simulink model "taskBasedWalking_legacy"  (Simulink 8.3)
settings: Solver=FixedStepDiscrete  StartTime=0.0  StopTime=Config.t_end  FixedStep=Config.t_step  RelTol=1e-3
InitFcn:
  | cd(fileparts(which(bdroot)));
  | initTaskBasedWalking;
StopFcn:
  | cd(fileparts(which(bdroot)));
  | stopTaskBasedWalking;
undefined symbols (not defined in the file): biasVectorConstraint_feet, Config, ConstraintMatrix_feet, DiscIntNeverNeededParam, Gains, ROBOT_DOF, Sat
libraries: WBToolboxLibrary x78
(part 2 of 3)

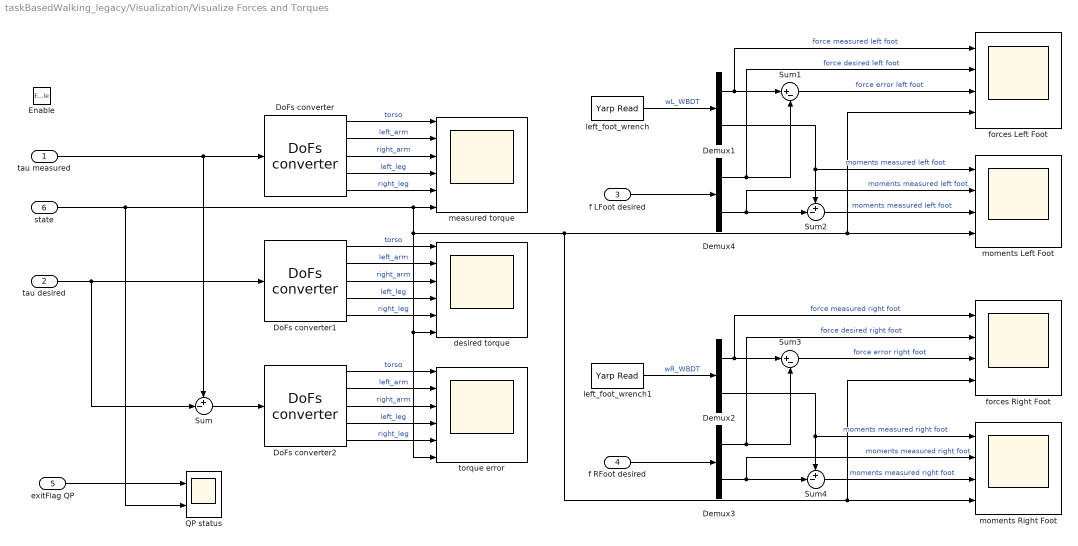
== system taskBasedWalking_legacy/Visualization/Visualize Forces and Torques ==
  tau measured : Inport
  tau desired : Inport  Port=2
  f LFoot desired : Inport  Port=3
  f RFoot desired : Inport  Port=4
  exitFlag QP : Inport  Port=5
  state : Inport  Port=6
  Enable : EnablePort
  Demux{1..4} (4 alike) : Demux  Outputs=[3;3]
  DoFs converter : WBToolboxLibrary/Utilities/DoFs converter  yarp2WBIOption=From YARP to WBI
  DoFs converter1 : WBToolboxLibrary/Utilities/DoFs converter  yarp2WBIOption=From YARP to WBI
  DoFs converter2 : WBToolboxLibrary/Utilities/DoFs converter  yarp2WBIOption=From YARP to WBI
  QP status : Scope  NumInputPorts=2
      settings: TimeRange=auto  MaxDataPoints=5000  SaveName=exitFlagQP_DATA  YMin=-1.00000~0.75  YMax=1.00000~3.25  SampleTime=-1
  Sum : Sum  Inputs=+-|
  Sum1 : Sum  Inputs=|+-
  Sum2 : Sum  Inputs=+-|
  Sum3 : Sum  Inputs=|+-
  Sum4 : Sum  Inputs=+-|
  desired torque : Scope  NumInputPorts=6
      settings: TimeRange=14  ShowLegends=on  MaxDataPoints=5000  SaveName=tauDes_DATA  YMin=-29.31633~-6.97567~-8.31868~-17.81518~-20.85132~0.75  YMax=21.22105~7.45092~10.09722~31.90811~36.21162~3.25  SampleTime=-1
  forces Left Foot : Scope  NumInputPorts=4
      settings: TimeRange=40  MaxDataPoints=5000  SaveName=LFoot_forces_DATA  YMin=-94.50547~-90.33374~-124.32192~0.75  YMax=380.58154~375.05705~119.64102~3.25  SampleTime=-1
  forces Right Foot : Scope  NumInputPorts=4
      settings: TimeRange=40  MaxDataPoints=5000  SaveName=RFoot_forces_DATA  YMin=-51.60497~-22.1975~-34.93363~0.9  YMax=197.58058~186.84107~13.61516~1.1  SampleTime=-1
  left_foot_wrench : WBToolboxLibrary/Utilities/Yarp Read  portName=Ports.LEFT_FOOT_EXT_WRENCH  signalSize=6  timeout=0.5  blocking=off  timestamp=off  autoconnect=on  errorOnConnection=on
  left_foot_wrench1 : WBToolboxLibrary/Utilities/Yarp Read  portName=Ports.RIGHT_FOOT_EXT_WRENCH  signalSize=6  timeout=0.5  blocking=off  timestamp=off  autoconnect=on  errorOnConnection=on
  measured torque : Scope  NumInputPorts=6
      settings: TimeRange=14  ShowLegends=on  MaxDataPoints=5000  SaveName=tauMeas_DATA  YMin=-11.47679~-4.18596~-4.23181~-18.73707~-21.78999~0.75  YMax=12.06319~6.82355~7.49283~33.43238~33.30445~3.25  SampleTime=-1
  moments Left Foot : Scope  NumInputPorts=4
      settings: TimeRange=40  ShowLegends=on  MaxDataPoints=5000  SaveName=LFoot_moments_DATA  YMin=-9.62259~-10.62436~-12.71673~0.75  YMax=14.01039~14.13793~13.77201~3.25  SampleTime=-1
  moments Right Foot : Scope  NumInputPorts=4
      settings: TimeRange=40  MaxDataPoints=5000  SaveName=RFoot_moments_DATA  YMin=-32.91586~-23.80001~-19.34028~0.75  YMax=21.19597~19.42571~23.95955~3.25  SampleTime=-1
  torque error : Scope  NumInputPorts=6
      settings: TimeRange=14  ShowLegends=on  MaxDataPoints=5000  SaveName=tauErr_DATA  YMin=-24.82167~-15.35375~-17.84626~-32.8437~-37.60868~0.75  YMax=19.17022~15.52326~18.81152~24.48279~21.81289~3.25  SampleTime=-1
  wires:
  Sum2/1 -> moments Left Foot/3  "moments measured left foot"
  state/1 -> QP status/2, torque error/6, desired torque/6, forces Right Foot/4, moments Right Foot/4, forces Left Foot/4, moments Left Foot/4, measured torque/6
  DoFs converter1/2 -> desired torque/2  "left_arm"
  Demux4/1 -> forces Left Foot/2, Sum1/2  "force desired left foot"
  DoFs converter2/1 -> torque error/1  "torso"
  DoFs converter1/4 -> desired torque/4  "left_leg"
  Demux4/2 -> moments Left Foot/2, Sum2/2  "moments measured left foot"
  DoFs converter/1 -> measured torque/1  "torso"
  DoFs converter2/3 -> torque error/3  "right_arm"
  f RFoot desired/1 -> Demux3/1
  DoFs converter1/1 -> desired torque/1  "torso"
  Sum4/1 -> moments Right Foot/3  "moments measured right foot"
  tau desired/1 -> Sum/2, DoFs converter1/1
  Demux2/1 -> forces Right Foot/1, Sum3/1  "force measured right foot"
  DoFs converter2/2 -> torque error/2  "left_arm"
  Sum3/1 -> forces Right Foot/3  "force error right foot"
  DoFs converter/5 -> measured torque/5  "right_leg"
  DoFs converter2/5 -> torque error/5  "right_leg"
  exitFlag QP/1 -> QP status/1
  left_foot_wrench/1 -> Demux1/1  "wL_WBDT"
  DoFs converter1/3 -> desired torque/3  "right_arm"
  Demux3/1 -> forces Right Foot/2, Sum3/2  "force desired right foot"
  f LFoot desired/1 -> Demux4/1
  Sum1/1 -> forces Left Foot/3  "force error left foot"
  tau measured/1 -> Sum/1, DoFs converter/1
  DoFs converter1/5 -> desired torque/5  "right_leg"
  DoFs converter/2 -> measured torque/2  "left_arm"
  DoFs converter/3 -> measured torque/3  "right_arm"
  Demux3/2 -> moments Right Foot/2, Sum4/2  "moments measured right foot"
  Sum/1 -> DoFs converter2/1
  Demux1/1 -> forces Left Foot/1, Sum1/1  "force measured left foot"
  DoFs converter/4 -> measured torque/4  "left_leg"
  Demux1/2 -> moments Left Foot/1, Sum2/1  "moments measured left foot"
  left_foot_wrench1/1 -> Demux2/1  "wR_WBDT"
  DoFs converter2/4 -> torque error/4  "left_leg"
  Demux2/2 -> moments Right Foot/1, Sum4/1  "moments measured right foot"

== system taskBasedWalking_legacy/Visualization/Visualize Gain Scheduling ==
  Kp_CoM : Inport
  Kd_CoM : Inport  Port=2
  Kp_LFoot : Inport  Port=3
  Kd_LFoot : Inport  Port=4
  Kp_RFoot : Inport  Port=5
  Kd_RFoot : Inport  Port=6
  Kp_rot_task : Inport  Port=7
  Kd_rot_task : Inport  Port=8
  impedances : Inport  Port=9
  dampings : Inport  Port=10
  state : Inport  Port=11
  Enable : EnablePort
  DoFs converter1 : WBToolboxLibrary/Utilities/DoFs converter  yarp2WBIOption=From YARP to WBI
  DoFs converter4 : WBToolboxLibrary/Utilities/DoFs converter  yarp2WBIOption=From YARP to WBI
  joint position gains : Scope  NumInputPorts=6
      settings: TimeRange=auto  MaxDataPoints=5000  SaveName=impedances_DATA  YMin=-10~-10~-10~-10~-10~-10  YMax=10~10~10~10~10~10  SampleTime=-1
  joint velocity gains : Scope  NumInputPorts=6
      settings: TimeRange=auto  MaxDataPoints=5000  SaveName=dampings_DATA  YMin=-1.00000~-1.00000~-1.00000~-1.00000~-1.00000~0.9  YMax=1.00000~1.00000~1.00000~1.00000~1.00000~1.1  SampleTime=-1
  orient gains rot task : Scope  NumInputPorts=2
      settings: TimeRange=auto  MaxDataPoints=5000  SaveName=Kp_rot_task_DATA  YMin=40.00000~0.75  YMax=60.00000~3.25  SampleTime=-1
  pos gains CoM : Scope  NumInputPorts=2
      settings: TimeRange=auto  MaxDataPoints=5000  SaveName=Kp_CoM_DATA  YMin=40.00000~0.75  YMax=60.00000~3.25  SampleTime=-1
  pose gains LFoot : Scope  NumInputPorts=2
      settings: TimeRange=auto  MaxDataPoints=5000  SaveName=Kp_LFoot_DATA  YMin=-9.375~0.75  YMax=834.375~3.25  SampleTime=-1
  pose gains RFoot : Scope  NumInputPorts=2
      settings: TimeRange=auto  MaxDataPoints=5000  SaveName=Kp_RFoot_DATA  YMin=-0.15075~0.9  YMax=0.68063~1.1  SampleTime=-1
  vel gains CoM : Scope  NumInputPorts=2
      settings: TimeRange=auto  MaxDataPoints=5000  SaveName=Kd_CoM_DATA  YMin=12.3762~0.625  YMax=15.10531~4.375  SampleTime=-1
  vel gains LFoot : Scope  NumInputPorts=2
      settings: TimeRange=auto  MaxDataPoints=5000  SaveName=Kd_LFoot_DATA  YMin=0.31598~0.75  YMax=1.48634~3.25  SampleTime=-1
  vel gains RFoot : Scope  NumInputPorts=2
      settings: TimeRange=auto  MaxDataPoints=5000  SaveName=Kd_RFoot_DATA  YMin=-0.15075~0.9  YMax=0.68063~1.1  SampleTime=-1
  vel gains rot task : Scope  NumInputPorts=2
      settings: TimeRange=auto  MaxDataPoints=5000  SaveName=Kd_rot_task_DATA  YMin=-0.15075~0.9  YMax=0.68063~1.1  SampleTime=-1
  wires:
  Kp_CoM/1 -> pos gains CoM/1
  Kp_LFoot/1 -> pose gains LFoot/1
  Kp_RFoot/1 -> pose gains RFoot/1
  Kp_rot_task/1 -> orient gains rot task/1
  state/1 -> vel gains LFoot/2, pose gains LFoot/2, vel gains CoM/2, vel gains rot task/2, orient gains rot task/2, vel gains RFoot/2, joint velocity gains/6, joint position gains/6, pose gains RFoot/2, pos gains CoM/2
  Kd_CoM/1 -> vel gains CoM/1
  Kd_LFoot/1 -> vel gains LFoot/1
  Kd_RFoot/1 -> vel gains RFoot/1
  Kd_rot_task/1 -> vel gains rot task/1
  DoFs converter4/2 -> joint position gains/2  "left_arm"
  DoFs converter4/1 -> joint position gains/1  "torso"
  DoFs converter4/4 -> joint position gains/4  "left_leg"
  DoFs converter4/3 -> joint position gains/3  "right_arm"
  DoFs converter4/5 -> joint position gains/5  "right_leg"
  DoFs converter1/2 -> joint velocity gains/2  "left_arm"
  DoFs converter1/1 -> joint velocity gains/1  "torso"
  DoFs converter1/4 -> joint velocity gains/4  "left_leg"
  DoFs converter1/3 -> joint velocity gains/3  "right_arm"
  DoFs converter1/5 -> joint velocity gains/5  "right_leg"
  impedances/1 -> DoFs converter4/1
  dampings/1 -> DoFs converter1/1

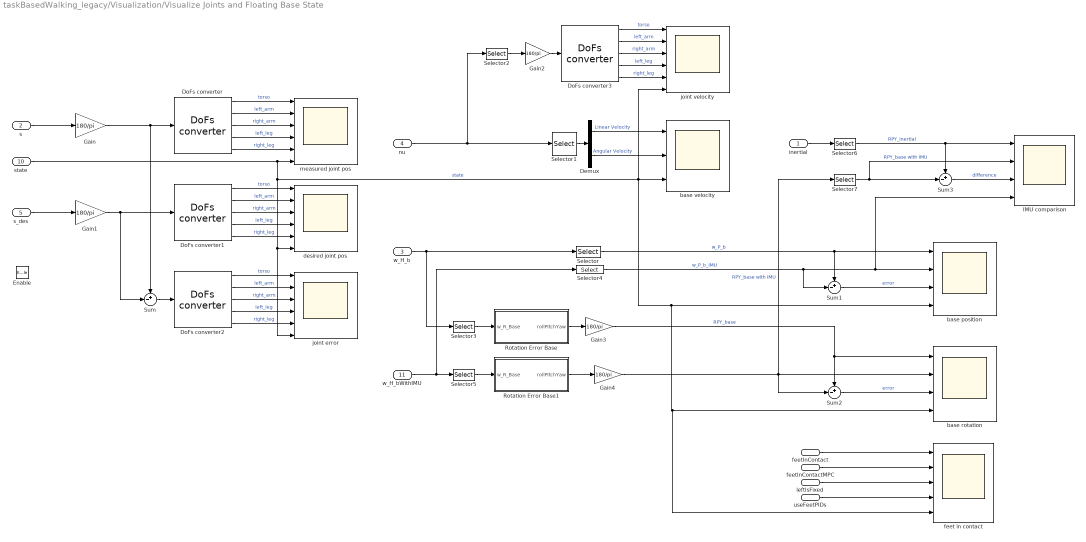
== system taskBasedWalking_legacy/Visualization/Visualize Joints and Floating Base State ==
  inertial : Inport
  s : Inport  Port=2
  w_H_b : Inport  Port=3
  nu : Inport  Port=4
  s_des : Inport  Port=5
  feetInContact : Inport  Port=6
  useFeetPIDs : Inport  Port=7
  feetInContactMPC : Inport  Port=8
  leftIsFixed : Inport  Port=9
  state : Inport  Port=10
  w_H_bWithIMU : Inport  Port=11
  Enable : EnablePort
  Demux : Demux  Outputs=2
  DoFs converter{,1..3} (4 alike) : WBToolboxLibrary/Utilities/DoFs converter  yarp2WBIOption=From YARP to WBI
  Gain{,1..4} (5 alike) : Gain  Gain=180/pi
  IMU comparison : Scope  NumInputPorts=4
      settings: TimeRange=auto  MaxDataPoints=5000  SaveToWorkspace=off  SaveName=ScopeData2  YMin=-12.46344~-15.58042~-22.96688~-0.21919  YMax=8.17339~13.72293~16.2002~0.70364  SampleTime=-1
  Rotation Error Base : Subsystem
  Rotation Error Base1 : Subsystem
  Selector : Selector  NumberOfDimensions=2  InputPortWidth=3  IndexOptions=Index vector (dialog),Index vector (dialog)  Indices=[1:3],4  OutputSizes=1,1
  Selector1 : Selector  InputPortWidth=ROBOT_DOF+6  IndexOptions=Index vector (dialog)  Indices=[1:6]  OutputSizes=1
  Selector2 : Selector  InputPortWidth=ROBOT_DOF+6  IndexOptions=Index vector (dialog)  Indices=[7:ROBOT_DOF+6]  OutputSizes=1
  Selector3 : Selector  NumberOfDimensions=2  InputPortWidth=3  IndexOptions=Index vector (dialog),Index vector (dialog)  Indices=[1:3],[1:3]  OutputSizes=1,1
  Selector4 : Selector  NumberOfDimensions=2  InputPortWidth=3  IndexOptions=Index vector (dialog),Index vector (dialog)  Indices=[1:3],4  OutputSizes=1,1
  Selector5 : Selector  NumberOfDimensions=2  InputPortWidth=3  IndexOptions=Index vector (dialog),Index vector (dialog)  Indices=[1:3],[1:3]  OutputSizes=1,1
  Selector6 : Selector  InputPortWidth=12  IndexOptions=Index vector (dialog)  Indices=[1:2]  OutputSizes=1
  Selector7 : Selector  InputPortWidth=3  IndexOptions=Index vector (dialog)  Indices=[1:2]  OutputSizes=1
  Sum{,1..3} (4 alike) : Sum  Inputs=+-|
  base position : Scope  NumInputPorts=4
      settings: TimeRange=auto  MaxDataPoints=5000  SaveName=basePos_DATA  YMin=-0.22398~-0.21941~-0.00771~0.75  YMax=0.95033~0.93824~0.00949~3.25  SampleTime=-1
  base rotation : Scope  NumInputPorts=4
      settings: TimeRange=auto  MaxDataPoints=5000  SaveName=BaseRotation_DATA  YMin=-224.99475~-224.99475~-4.20767~0.75  YMax=224.99655~224.99655~2.37208~3.25  SampleTime=-1
  base velocity : Scope  NumInputPorts=3
      settings: TimeRange=auto  ShowLegends=on  MaxDataPoints=5000  SaveName=baseVel_DATA  YMin=-0.22618~-0.79944~0.75  YMax=0.42394~0.82635~3.25  SampleTime=-1
  desired joint pos : Scope  NumInputPorts=6
      settings: TimeRange=auto  ShowLegends=on  MaxDataPoints=5000  SaveName=jointDes_DATA  YMin=-6.59451~-23.74816~-24.05925~-41.17118~-41.50525~0.75  YMax=12.61384~48.08227~47.96861~18.71413~18.81596~3.25  SampleTime=-1
  feet in contact : Scope  NumInputPorts=5
      settings: TimeRange=auto  ShowLegends=on  MaxDataPoints=5000  SaveName=feetInContact_DATA  YMin=0.9~0.9~-1.00000~-0.125~0.9  YMax=1.1~1.1~1.00000~1.125~1.1  SampleTime=-1
  joint error : Scope  NumInputPorts=6
      settings: TimeRange=auto  ShowLegends=on  MaxDataPoints=5000  SaveName=jointErr_DATA  YMin=-13.39791~-5.05479~-5.63796~-13.82698~-9.31683~0.75  YMax=10.2644~7.99929~9.10191~9.60583~15.76566~3.25  SampleTime=-1
  joint velocity : Scope  NumInputPorts=6
      settings: TimeRange=auto  MaxDataPoints=5000  SaveName=jointVel_DATA  YMin=-65.10651~-223.32925~-75.18237~-29.76616~-17.38591~0.9  YMax=57.73467~97.18392~97.27593~28.94218~48.25756~1.1  SampleTime=-1
  measured joint pos : Scope  NumInputPorts=6
      settings: TimeRange=auto  MaxDataPoints=5000  SaveName=jointMeas_DATA  YMin=-3.77381~-21.81821~-14.09343~-38.97066~-38.66716~0.9  YMax=13.63956~37.00685~38.07115~10.81813~10.33885~1.1  SampleTime=-1
  wires:
  DoFs converter1/2 -> desired joint pos/2  "left_arm"
  DoFs converter/5 -> measured joint pos/5  "right_leg"
  DoFs converter2/1 -> joint error/1  "torso"
  DoFs converter/4 -> measured joint pos/4  "left_leg"
  DoFs converter/2 -> measured joint pos/2  "left_arm"
  s/1 -> Gain/1
  DoFs converter1/1 -> desired joint pos/1  "torso"
  DoFs converter1/4 -> desired joint pos/4  "left_leg"
  DoFs converter1/3 -> desired joint pos/3  "right_arm"
  DoFs converter/3 -> measured joint pos/3  "right_arm"
  DoFs converter2/5 -> joint error/5  "right_leg"
  DoFs converter2/2 -> joint error/2  "left_arm"
  DoFs converter/1 -> measured joint pos/1  "torso"
  s_des/1 -> Gain1/1
  DoFs converter1/5 -> desired joint pos/5  "right_leg"
  DoFs converter2/4 -> joint error/4  "left_leg"
  Sum/1 -> DoFs converter2/1
  DoFs converter2/3 -> joint error/3  "right_arm"
  DoFs converter3/5 -> joint velocity/5  "right_leg"
  DoFs converter3/1 -> joint velocity/1  "torso"
  DoFs converter3/4 -> joint velocity/4  "left_leg"
  DoFs converter3/3 -> joint velocity/3  "right_arm"
  DoFs converter3/2 -> joint velocity/2  "left_arm"
  nu/1 -> Selector2/1, Selector1/1
  w_H_b/1 -> Selector3/1, Selector/1
  Gain/1 -> Sum/1, DoFs converter/1
  Gain1/1 -> Sum/2, DoFs converter1/1
  Gain2/1 -> DoFs converter3/1
  Selector/1 -> base position/1, Sum1/1  "w_P_b"
  Selector2/1 -> Gain2/1
  state/1 -> measured joint pos/6, feet in contact/5, base rotation/4, base position/4, base velocity/3, joint velocity/6, joint error/6, desired joint pos/6  "state"
  Selector1/1 -> Demux/1
  feetInContact/1 -> feet in contact/1
  Rotation Error Base/1(rollPitchYaw) -> Gain3/1
  Gain3/1 -> Sum2/1, base rotation/1  "RPY_base"
  feetInContactMPC/1 -> feet in contact/2
  leftIsFixed/1 -> feet in contact/3
  useFeetPIDs/1 -> feet in contact/4
  Selector3/1 -> Rotation Error Base/1(w_R_Base)
  w_H_bWithIMU/1 -> Selector4/1, Selector5/1
  Selector4/1 -> Sum1/2, IMU comparison/4, base position/2  "w_P_b_IMU"
  Selector5/1 -> Rotation Error Base1/1(w_R_Base)
  Rotation Error Base1/1(rollPitchYaw) -> Gain4/1
  Sum1/1 -> base position/3  "error"
  Gain4/1 -> Selector7/1, base rotation/2, Sum2/2  "RPY_base with IMU"
  Sum2/1 -> base rotation/3  "error"
  inertial/1 -> Selector6/1
  Selector6/1 -> Sum3/1, IMU comparison/1  "RPY_inertial"
  Sum3/1 -> IMU comparison/3  "difference"
  Selector7/1 -> IMU comparison/2, Sum3/2  "RPY_base with IMU"
  Demux/1 -> base velocity/1  "Linear Velocity"
  Demux/2 -> base velocity/2  "Angular Velocity"

== system taskBasedWalking_legacy/Visualization/Visualize Smoothing (orientation) ==
  w_R_LFoot_des : Inport
  w_R_RFoot_des : Inport  Port=2
  w_R_rot_task_des : Inport  Port=3
  w_R_LFoot : Inport  Port=4
  w_R_RFoot : Inport  Port=5
  w_R_rot_task : Inport  Port=6
  V_base : Inport  Port=7
  VDot_base : Inport  Port=8
  Enable : EnablePort
  Demux : Demux  Outputs=3
  Demux1 : Demux  Outputs=3
  Demux2 : Demux  Outputs=3
  Gain : Gain  Gain=180/pi
  Gain1 : Gain  Gain=180/pi
  Gain2 : Gain  Gain=180/pi
  Rotation Error LFoot : Scope  NumInputPorts=3
      settings: TimeRange=auto  MaxDataPoints=5000  SaveName=SmootingLFoot_error_DATA  YMin=-0.000000000000000031~0.0000000000000002~-0.00000000000000006  YMax=0.000000000000000048~0.0000000000000052~0.00000000000000012  SampleTime=-1
  Rotation Error Left Foot : Subsystem
  Rotation Error RFoot : Scope  NumInputPorts=3
      settings: TimeRange=auto  ShowLegends=on  MaxDataPoints=5000  SaveName=SmootingRFoot_error_DATA  YMin=-0.04233~-0.55929~-0.07094  YMax=0.38093~0.06214~0.041  SampleTime=-1
  Rotation Error Right Foot : Subsystem
  Rotation Error Rot Task : Subsystem
  Rotation Error Rotational Task : Scope  NumInputPorts=3
      settings: TimeRange=auto  MaxDataPoints=5000  SaveName=Smooting_rot_task_error_DATA  YMin=-0.00000000000000527~0.00000000000000017539~0.000000000000000046  YMax=-0.00000000000000477~0.00000000000000017588~0.000000000000000066  SampleTime=-1
  stability of base smoothing : Scope  NumInputPorts=2
      settings: TimeRange=auto  MaxDataPoints=5000  SaveName=smoothBaseStability_DATA  YMin=-0.00125~-0.10529  YMax=0.01038~0.0117  SampleTime=-1
  wires:
  w_R_LFoot/1 -> Rotation Error Left Foot/1(w_R_LFoot)
  w_R_LFoot_des/1 -> Rotation Error Left Foot/2(w_R_LFoot_des)
  Rotation Error Left Foot/1(rollPitchYaw) -> Gain/1
  Demux/1 -> Rotation Error LFoot/1  "roll"
  Demux/2 -> Rotation Error LFoot/2  "pitch"
  Demux/3 -> Rotation Error LFoot/3  "yaw"
  w_R_RFoot/1 -> Rotation Error Right Foot/1(w_R_RFoot)
  w_R_RFoot_des/1 -> Rotation Error Right Foot/2(w_R_RFoot_des)
  Rotation Error Right Foot/1(rollPitchYaw) -> Gain1/1
  Demux1/1 -> Rotation Error RFoot/1  "roll"
  Demux1/2 -> Rotation Error RFoot/2  "pitch"
  Demux1/3 -> Rotation Error RFoot/3  "yaw"
  w_R_rot_task/1 -> Rotation Error Rot Task/1(w_R_rot_task)
  w_R_rot_task_des/1 -> Rotation Error Rot Task/2(w_R_rot_task_des)
  Rotation Error Rot Task/1(rollPitchYaw) -> Gain2/1
  Demux2/1 -> Rotation Error Rotational Task/1  "roll"
  Demux2/2 -> Rotation Error Rotational Task/2  "pitch"
  Demux2/3 -> Rotation Error Rotational Task/3  "yaw"
  Gain/1 -> Demux/1
  Gain1/1 -> Demux1/1
  Gain2/1 -> Demux2/1
  V_base/1 -> stability of base smoothing/1
  VDot_base/1 -> stability of base smoothing/2

== system taskBasedWalking_legacy/synchronizer/GAZEBO_SYNCHRONIZER ==
  Enable : EnablePort
  Simulator Synchronizer : WBToolboxLibrary/Utilities/Simulator Synchronizer  period=Config.t_step  serverPortName='/clock/rpc'  clientPortName='/WBT_synchronizer/rpc:o'

== system taskBasedWalking_legacy/synchronizer/REAL_TIME_SYNC ==
  Enable : EnablePort
  Real Time Synchronizer : WBToolboxLibrary/Utilities/Real Time Synchronizer  period=Config.t_step

== system taskBasedWalking_legacy/Dynamics and Kinematics/Compute Dynamic and Kinematic Quantities/Jacobians and JDot_nu ==
  s : Inport
  nu_b : Inport  Port=2
  sDot : Inport  Port=3
  w_H_b : Inport  Port=4
  DotJ Nu CoM : WBToolboxLibrary/wholeBodyModel/Jacobians/DotJ Nu  frameName=Frames.COM
  DotJ Nu LFoot : WBToolboxLibrary/wholeBodyModel/Jacobians/DotJ Nu  frameName=Frames.LEFT_FOOT
  DotJ Nu RFoot : WBToolboxLibrary/wholeBodyModel/Jacobians/DotJ Nu  frameName=Frames.RIGHT_FOOT
  DotJ Nu rotational task : WBToolboxLibrary/wholeBodyModel/Jacobians/DotJ Nu  frameName=Frames.ROT_TASK_LINK
  Jacobian CoM : WBToolboxLibrary/wholeBodyModel/Jacobians/Jacobian  frameName=Frames.COM
  Jacobian LFoot : WBToolboxLibrary/wholeBodyModel/Jacobians/Jacobian  frameName=Frames.LEFT_FOOT
  Jacobian RFoot : WBToolboxLibrary/wholeBodyModel/Jacobians/Jacobian  frameName=Frames.RIGHT_FOOT
  Jacobian rotational task : WBToolboxLibrary/wholeBodyModel/Jacobians/Jacobian  frameName=Frames.ROT_TASK_LINK
  J_LFoot : Outport
  J_RFoot : Outport  Port=2
  J_CoM : Outport  Port=3
  J_rot_task : Outport  Port=4
  JDot_nu_LFoot : Outport  Port=5
  JDot_nu_RFoot : Outport  Port=6
  JDot_nu_CoM : Outport  Port=7
  JDot_nu_rot_task : Outport  Port=8
  wires:
  Jacobian CoM/1 -> J_CoM/1
  Jacobian rotational task/1 -> J_rot_task/1
  Jacobian LFoot/1 -> J_LFoot/1
  Jacobian RFoot/1 -> J_RFoot/1
  w_H_b/1 -> Jacobian RFoot/1, Jacobian LFoot/1, DotJ Nu RFoot/1, DotJ Nu LFoot/1, DotJ Nu rotational task/1, DotJ Nu CoM/1, Jacobian CoM/1, Jacobian rotational task/1
  sDot/1 -> DotJ Nu RFoot/4, DotJ Nu LFoot/4, DotJ Nu rotational task/4, DotJ Nu CoM/4
  nu_b/1 -> DotJ Nu CoM/3, DotJ Nu RFoot/3, DotJ Nu LFoot/3, DotJ Nu rotational task/3
  s/1 -> DotJ Nu RFoot/2, DotJ Nu LFoot/2, DotJ Nu rotational task/2, DotJ Nu CoM/2, Jacobian RFoot/2, Jacobian CoM/2, Jacobian rotational task/2, Jacobian LFoot/2
  DotJ Nu RFoot/1 -> JDot_nu_RFoot/1
  DotJ Nu LFoot/1 -> JDot_nu_LFoot/1
  DotJ Nu rotational task/1 -> JDot_nu_rot_task/1
  DotJ Nu CoM/1 -> JDot_nu_CoM/1

== system taskBasedWalking_legacy/Dynamics and Kinematics/Compute Dynamic and Kinematic Quantities/Mass Matrix and Bias Forces ==
  s : Inport
  nu_b : Inport  Port=2
  sDot : Inport  Port=3
  w_H_b : Inport  Port=4
  Add motors reflected inertias : Subsystem
  Get Bias Forces : WBToolboxLibrary/wholeBodyModel/Dynamics/Get Bias Forces
  Mass Matrix : WBToolboxLibrary/wholeBodyModel/Dynamics/Mass Matrix
  h(q,nu) : Outport
  M(q) : Outport  Port=2
  wires:
  w_H_b/1 -> Mass Matrix/1, Get Bias Forces/1
  s/1 -> Mass Matrix/2, Get Bias Forces/2
  sDot/1 -> Get Bias Forces/4
  nu_b/1 -> Get Bias Forces/3
  Get Bias Forces/1 -> h(q,nu)/1
  Mass Matrix/1 -> Add motors reflected inertias/1(M)
  Add motors reflected inertias/1(M_with_motor_inertia) -> M(q)/1

== system taskBasedWalking_legacy/Dynamics and Kinematics/Compute Tasks Accelerations/ComputeTasksPoseAndVelocity ==
  J_LFoot : Inport
  J_RFoot : Inport  Port=2
  J_CoM : Inport  Port=3
  J_rot_task : Inport  Port=4
  s : Inport  Port=5
  w_H_b : Inport  Port=6
  nu : Inport  Port=7
  Compose Task Pose and Velocity : MATLAB Function  TreatAsAtomicUnit=on
      settings: PermitHierarchicalResolution=ParametersOnly
  Product{,1..3} (4 alike) : Product  Multiplication=Matrix(*)
  Task position and orientation : Subsystem
  pos_vel_CoM : Outport
  pose_vel_LFoot : Outport  Port=2
  pose_vel_RFoot : Outport  Port=3
  orient_vel_rot_task : Outport  Port=4
  w_H_l_sole : Outport  Port=5
  w_H_r_sole : Outport  Port=6
  wires:
  Compose Task Pose and Velocity/3(pose_vel_RFoot) -> pose_vel_RFoot/1
  Compose Task Pose and Velocity/2(pose_vel_LFoot) -> pose_vel_LFoot/1
  Compose Task Pose and Velocity/1(pos_vel_CoM) -> pos_vel_CoM/1
  Compose Task Pose and Velocity/4(orient_vel_rot_task) -> orient_vel_rot_task/1
  nu/1 -> Product1/2, Product/2, Product2/2, Product3/2
  J_rot_task/1 -> Product3/1
  Product/1 -> Compose Task Pose and Velocity/1(vel_CoM)
  Product1/1 -> Compose Task Pose and Velocity/2(vel_LFoot)
  Product2/1 -> Compose Task Pose and Velocity/3(vel_RFoot)
  Product3/1 -> Compose Task Pose and Velocity/4(vel_rot_task)
  s/1 -> Task position and orientation/1(s)
  w_H_b/1 -> Task position and orientation/2(w_H_b)
  Task position and orientation/1(w_H_CoM) -> Compose Task Pose and Velocity/5(w_H_CoM)
  Task position and orientation/2(w_H_l_sole) -> w_H_l_sole/1, Compose Task Pose and Velocity/6(w_H_l_sole)
  Task position and orientation/3(w_H_r_sole) -> w_H_r_sole/1, Compose Task Pose and Velocity/7(w_H_r_sole)
  Task position and orientation/4(w_H_rot_task) -> Compose Task Pose and Velocity/8(w_H_rot_task)
  J_RFoot/1 -> Product2/1
  J_LFoot/1 -> Product1/1
  J_CoM/1 -> Product/1

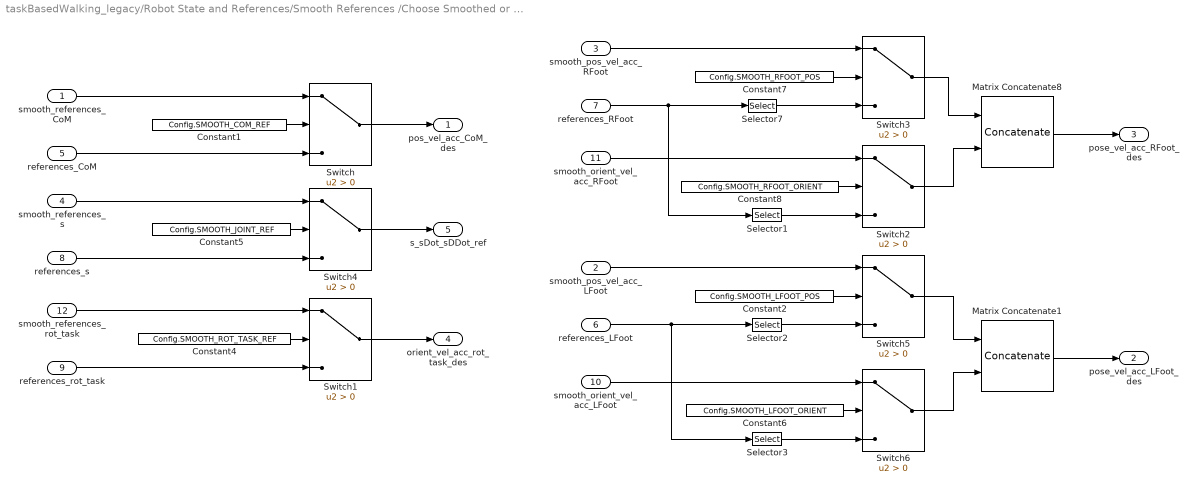
== system taskBasedWalking_legacy/Robot State and References/Smooth References /Choose Smoothed or Direct References ==
  smooth_references_CoM : Inport
  smooth_pos_vel_acc_LFoot : Inport  Port=2
  smooth_pos_vel_acc_RFoot : Inport  Port=3
  smooth_references_s : Inport  Port=4
  references_CoM : Inport  Port=5
  references_LFoot : Inport  Port=6
  references_RFoot : Inport  Port=7
  references_s : Inport  Port=8
  references_rot_task : Inport  Port=9
  smooth_orient_vel_acc_LFoot : Inport  Port=10
  smooth_orient_vel_acc_RFoot : Inport  Port=11
  smooth_references_rot_task : Inport  Port=12
  Constant1 : Constant  Value=Config.SMOOTH_COM_REF
  Constant2 : Constant  Value=Config.SMOOTH_LFOOT_POS
  Constant4 : Constant  Value=Config.SMOOTH_ROT_TASK_REF
  Constant5 : Constant  Value=Config.SMOOTH_JOINT_REF
  Constant6 : Constant  Value=Config.SMOOTH_LFOOT_ORIENT
  Constant7 : Constant  Value=Config.SMOOTH_RFOOT_POS
  Constant8 : Constant  Value=Config.SMOOTH_RFOOT_ORIENT
  Matrix Concatenate1 : Concatenate  Mode=Multidimensional array
  Matrix Concatenate8 : Concatenate  Mode=Multidimensional array
  Selector1 : Selector  NumberOfDimensions=2  InputPortWidth=ROBOT_DOF  IndexOptions=Index vector (dialog),Index vector (dialog)  Indices=[4:6],[1:5]  OutputSizes=1,1
  Selector2 : Selector  NumberOfDimensions=2  InputPortWidth=ROBOT_DOF  IndexOptions=Index vector (dialog),Index vector (dialog)  Indices=[1:3],[1:5]  OutputSizes=1,1
  Selector3 : Selector  NumberOfDimensions=2  InputPortWidth=ROBOT_DOF  IndexOptions=Index vector (dialog),Index vector (dialog)  Indices=[4:6],[1:5]  OutputSizes=1,1
  Selector7 : Selector  NumberOfDimensions=2  InputPortWidth=ROBOT_DOF  IndexOptions=Index vector (dialog),Index vector (dialog)  Indices=[1:3],[1:5]  OutputSizes=1,1
  Switch{,1..6} (7 alike) : Switch  Criteria=u2 > Threshold
  pos_vel_acc_CoM_des : Outport
  pose_vel_acc_LFoot_des : Outport  Port=2
  pose_vel_acc_RFoot_des : Outport  Port=3
  orient_vel_acc_rot_task_des : Outport  Port=4
  s_sDot_sDDot_ref : Outport  Port=5
  wires:
  Constant1/1 -> Switch/2
  Switch/1 -> pos_vel_acc_CoM_des/1
  Constant5/1 -> Switch4/2
  Switch4/1 -> s_sDot_sDDot_ref/1
  references_CoM/1 -> Switch/3
  smooth_references_CoM/1 -> Switch/1
  smooth_references_s/1 -> Switch4/1
  references_s/1 -> Switch4/3
  smooth_references_rot_task/1 -> Switch1/1
  references_rot_task/1 -> Switch1/3
  Constant4/1 -> Switch1/2
  Switch1/1 -> orient_vel_acc_rot_task_des/1
  smooth_pos_vel_acc_RFoot/1 -> Switch3/1
  Constant7/1 -> Switch3/2
  references_RFoot/1 -> Selector1/1, Selector7/1
  Selector7/1 -> Switch3/3
  smooth_orient_vel_acc_RFoot/1 -> Switch2/1
  Constant8/1 -> Switch2/2
  Selector1/1 -> Switch2/3
  Switch3/1 -> Matrix Concatenate8/1
  Switch2/1 -> Matrix Concatenate8/2
  references_LFoot/1 -> Selector3/1, Selector2/1
  Matrix Concatenate8/1 -> pose_vel_acc_RFoot_des/1
  Constant6/1 -> Switch6/2
  Matrix Concatenate1/1 -> pose_vel_acc_LFoot_des/1
  Switch5/1 -> Matrix Concatenate1/1
  Switch6/1 -> Matrix Concatenate1/2
  Constant2/1 -> Switch5/2
  Selector2/1 -> Switch5/3
  smooth_pos_vel_acc_LFoot/1 -> Switch5/1
  smooth_orient_vel_acc_LFoot/1 -> Switch6/1
  Selector3/1 -> Switch6/3

== system taskBasedWalking_legacy/Robot State and References/Smooth References /Smooth Reference Orientations ==
  w_R_LFoot_des : Inport
  w_R_RFoot_des : Inport  Port=2
  w_R_Rot_task_des : Inport  Port=3
  state : Inport  Port=4
  Compose Smoothed References : Subsystem
  Compute Smoothed Ref Orientations : Subsystem
  Constant{,1..5} (6 alike) : Constant  Value=zeros(3,1)
  smooth_orient_vel_acc_LFoot : Outport
  smooth_orient_vel_acc_RFoot : Outport  Port=2
  smooth_orient_vel_acc_Rot_task : Outport  Port=3
  wires:
  w_R_LFoot_des/1 -> Compute Smoothed Ref Orientations/1(w_R_LFoot_des)
  w_R_RFoot_des/1 -> Compute Smoothed Ref Orientations/2(w_R_RFoot_des)
  w_R_Rot_task_des/1 -> Compute Smoothed Ref Orientations/3(w_R_rot_task_des)
  Compute Smoothed Ref Orientations/3(w_R_LFoot) -> Compose Smoothed References/6(w_R_LFoot)
  Compute Smoothed Ref Orientations/2(w_R_RFoot) -> Compose Smoothed References/5(w_R_RFoot)
  Compute Smoothed Ref Orientations/1(w_R_rot_task) -> Compose Smoothed References/4(w_R_rot_task)
  Compose Smoothed References/1(orient_vel_acc_LFoot_des) -> smooth_orient_vel_acc_LFoot/1
  Compose Smoothed References/2(orient_vel_acc_RFoot_des) -> smooth_orient_vel_acc_RFoot/1
  Compose Smoothed References/3(orient_vel_acc_rot_task_des) -> smooth_orient_vel_acc_Rot_task/1
  state/1 -> Compute Smoothed Ref Orientations/4(state)
  Constant/1 -> Compose Smoothed References/1(omegaDot_LFoot)
  Constant1/1 -> Compose Smoothed References/2(omegaDot_RFoot)
  Constant2/1 -> Compose Smoothed References/3(omegaDot_rot_task)
  Constant5/1 -> Compose Smoothed References/9(omega_rot_task)
  Constant4/1 -> Compose Smoothed References/8(omega_RFoot)
  Constant3/1 -> Compose Smoothed References/7(omega_LFoot)

== system taskBasedWalking_legacy/Robot State and References/Smooth References /Smooth Reference Positions ==
  pos_CoM_des : Inport
  pos_LFoot_des : Inport  Port=2
  pos_RFoot_des : Inport  Port=3
  s_des : Inport  Port=4
  state : Inport  Port=5
  Configure Settling Times : MATLAB Function  TreatAsAtomicUnit=on
      settings: PermitHierarchicalResolution=ParametersOnly
  Matrix Concatenate1 : Concatenate  NumInputs=3  Mode=Multidimensional array  ConcatenateDimension=2
  Matrix Concatenate2 : Concatenate  NumInputs=4  Mode=Multidimensional array  ConcatenateDimension=2
  Matrix Concatenate3 : Concatenate  NumInputs=4  Mode=Multidimensional array  ConcatenateDimension=2
  Matrix Concatenate4 : Concatenate  NumInputs=3  Mode=Multidimensional array  ConcatenateDimension=2
  Minimum Jerk Trajectory Generator{,1..3} (4 alike) : WBToolboxLibrary/Utilities/Minimum Jerk Trajectory Generator  externalSettlingTime=on  settlingTime=3  sampleTime=Config.t_step  resetOnSettlingTime=off  firstDerivatives=on  secondDerivatives=on  explicitInitialValue=off
  Settling time1 : Constant  Value=zeros(3,2)
  smooth_references_CoM : Outport
  smooth_pos_vel_acc_LFoot : Outport  Port=2
  smooth_pos_vel_acc_RFoot : Outport  Port=3
  smooth_references_s : Outport  Port=4
  wires:
  Minimum Jerk Trajectory Generator2/2 -> Matrix Concatenate3/2
  pos_LFoot_des/1 -> Minimum Jerk Trajectory Generator2/1
  pos_RFoot_des/1 -> Minimum Jerk Trajectory Generator3/1
  Minimum Jerk Trajectory Generator2/3 -> Matrix Concatenate3/3
  Minimum Jerk Trajectory Generator2/1 -> Matrix Concatenate3/1
  Minimum Jerk Trajectory Generator1/3 -> Matrix Concatenate1/3
  Matrix Concatenate1/1 -> smooth_references_s/1
  Matrix Concatenate4/1 -> smooth_references_CoM/1
  Minimum Jerk Trajectory Generator1/1 -> Matrix Concatenate1/1
  pos_CoM_des/1 -> Minimum Jerk Trajectory Generator/1
  Minimum Jerk Trajectory Generator/3 -> Matrix Concatenate4/3
  Minimum Jerk Trajectory Generator/2 -> Matrix Concatenate4/2
  Minimum Jerk Trajectory Generator1/2 -> Matrix Concatenate1/2
  Minimum Jerk Trajectory Generator3/3 -> Matrix Concatenate2/3
  Matrix Concatenate3/1 -> smooth_pos_vel_acc_LFoot/1
  Matrix Concatenate2/1 -> smooth_pos_vel_acc_RFoot/1
  Minimum Jerk Trajectory Generator/1 -> Matrix Concatenate4/1
  Minimum Jerk Trajectory Generator3/2 -> Matrix Concatenate2/2
  s_des/1 -> Minimum Jerk Trajectory Generator1/1
  Settling time1/1 -> Matrix Concatenate2/4, Matrix Concatenate3/4
  Minimum Jerk Trajectory Generator3/1 -> Matrix Concatenate2/1
  state/1 -> Configure Settling Times/1(state)
  Configure Settling Times/1(smoothingTime_CoM) -> Minimum Jerk Trajectory Generator/2
  Configure Settling Times/2(smoothingTime_joints) -> Minimum Jerk Trajectory Generator1/2
  Configure Settling Times/3(smoothingTime_LFoot) -> Minimum Jerk Trajectory Generator2/2
  Configure Settling Times/4(smoothingTime_RFoot) -> Minimum Jerk Trajectory Generator3/2

== system taskBasedWalking_legacy/Robot State and References/State Machine/Compute State Velocity ==
  s : Inport
  w_H_b : Inport  Port=2
  "feetInContact " : Inport  Port=3
  BaseVelocitySmoothed : Inport  Port=4
  omega_world : Inport  Port=5
  Compute Base Velocity : MATLAB Function  TreatAsAtomicUnit=on
      settings: PermitHierarchicalResolution=ParametersOnly
  Constant : Constant  Value=Config.SMOOTH_BASE_VEL
  Demux : Demux  Outputs=[3,2,1]
  Feet Jacobians : Subsystem
  Get Measurement : WBToolboxLibrary/wholeBodyStates/Get Measurement  measuredType=Joints Velocity
  Mux : Mux  Inputs=2
  Mux1 : Mux  Inputs=[3,2,1]
  Mux2 : Mux  Inputs=2
  Scope : Scope  NumInputPorts=3
      settings: TimeRange=auto  MaxDataPoints=5000  SaveToWorkspace=off  YMin=-0.95609~-0.79944~-0.89123  YMax=0.96739~0.82635~0.93343  SampleTime=-1
  Scope1 : Scope  NumInputPorts=3
      settings: TimeRange=auto  MaxDataPoints=5000  SaveToWorkspace=off  SaveName=ScopeData2  YMin=-0.20959~-0.50156~-0.33817  YMax=0.19902~0.43295~0.56838  SampleTime=-1
  Selector : Selector  InputPortWidth=3  IndexOptions=Index vector (dialog)  Indices=3  OutputSizes=1
  Selector1 : Selector  InputPortWidth=3  IndexOptions=Index vector (dialog)  Indices=3  OutputSizes=1
  Selector2 : Selector  InputPortWidth=3  IndexOptions=Index vector (dialog)  Indices=[1:2]  OutputSizes=1
  Selector3 : Selector  InputPortWidth=3  IndexOptions=Index vector (dialog)  Indices=[3]  OutputSizes=1
  Sum : Sum  Inputs=+-|
  Sum1 : Sum  Inputs=+-|
  Switch : Switch  Criteria=u2 > Threshold
  nu : Outport
  wires:
  Mux/1 -> nu/1
  s/1 -> Feet Jacobians/1(s)
  w_H_b/1 -> Feet Jacobians/2(w_H_b)
  Feet Jacobians/1(J_LFoot) -> Compute Base Velocity/1(J_LeftFoot)
  Feet Jacobians/2(J_RFoot) -> Compute Base Velocity/2(J_RightFoot)
  Switch/1 -> Mux/1
  Constant/1 -> Switch/2
  BaseVelocitySmoothed/1 -> Switch/1
  Compute Base Velocity/1(nu_b) -> Demux/1
  Get Measurement/1 -> Compute Base Velocity/4(sDot), Mux/2
  Mux1/1 -> Switch/3
  Demux/1 -> Mux1/1
  Mux2/1 -> Scope/1, Selector/1, Sum/1  "omega kin"
  omega_world/1 -> Sum/2, Scope/2, Selector1/1, Selector3/1, Selector2/1  "omega imu"
  Sum/1 -> Scope/3  "diff"
  Selector/1 -> Sum1/1, Scope1/1  "yaw kin"
  Selector1/1 -> Scope1/2, Sum1/2  "yaw imu"
  Sum1/1 -> Scope1/3  "yaw diff"
  "feetInContact "/1 -> Compute Base Velocity/3(feetInContact)
  Selector2/1 -> Mux1/2
  Demux/3 -> Mux1/3, Mux2/2
  Demux/2 -> Mux2/1  "omega kin"

== system taskBasedWalking_legacy/Robot State and References/State Machine/Compute Transformation Matrices ==
  s : Inport
  IMU port : Inport  Port=2
  pos_quat_LFoot (MPC) : Inport  Port=3
  LFoot_is_fixed (MPC) : Inport  Port=4
  "pos_quat_RFoot (MPC) " : Inport  Port=5
  Compute Feet to Base Link Transforms : Subsystem
  Compute Fixed Foot to World Transform (MPC) : Subsystem
  w_walking_H_LFoot : Outport
  w_walking_H_RFoot : Outport  Port=2
  w_walking_H_b_initial : Outport  Port=3
  "b_H_LFoot " : Outport  Port=4
  b_H_RFoot : Outport  Port=5
  LFoot_is_fixed(MPC) : Outport  Port=6
  wires:
  IMU port/1 -> Compute Feet to Base Link Transforms/1(IMU port)
  s/1 -> Compute Feet to Base Link Transforms/2(s)
  "pos_quat_RFoot (MPC) "/1 -> Compute Fixed Foot to World Transform (MPC)/3("pos_quat_RFoot (MPC) ")
  LFoot_is_fixed (MPC)/1 -> Compute Fixed Foot to World Transform (MPC)/1(LFoot_is_fixed (MPC)), LFoot_is_fixed(MPC)/1
  pos_quat_LFoot (MPC)/1 -> Compute Fixed Foot to World Transform (MPC)/2(pos_quat_LFoot (MPC))
  Compute Feet to Base Link Transforms/1(b_H_LFoot) -> Compute Fixed Foot to World Transform (MPC)/4(b_H_LFoot), "b_H_LFoot "/1
  Compute Feet to Base Link Transforms/2(b_H_RFoot) -> Compute Fixed Foot to World Transform (MPC)/5(b_H_RFoot), b_H_RFoot/1
  Compute Fixed Foot to World Transform (MPC)/1(w_walking_H_b_initial) -> w_walking_H_b_initial/1
  Compute Fixed Foot to World Transform (MPC)/2(w_walking_H_LFoot) -> w_walking_H_LFoot/1
  Compute Fixed Foot to World Transform (MPC)/3(w_walking_H_RFoot) -> w_walking_H_RFoot/1

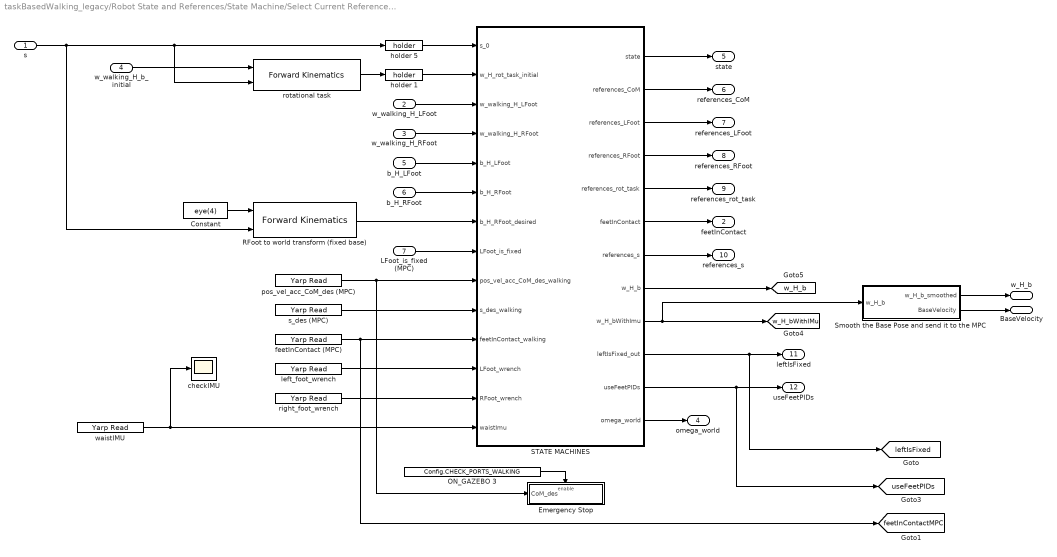
== system taskBasedWalking_legacy/Robot State and References/State Machine/Select Current References and Estimate w_H_b ==
  s : Inport
  w_walking_H_LFoot : Inport  Port=2
  w_walking_H_RFoot : Inport  Port=3
  w_walking_H_b_initial : Inport  Port=4
  b_H_LFoot : Inport  Port=5
  b_H_RFoot : Inport  Port=6
  LFoot_is_fixed (MPC) : Inport  Port=7
  Constant : Constant  Value=eye(4)
  Emergency Stop : Subsystem
  ON_GAZEBO 3 : Constant  Value=Config.CHECK_PORTS_WALKING
  RFoot to world transform (fixed base) : WBToolboxLibrary/wholeBodyModel/Kinematics/Forward Kinematics  frameName=Frames.RIGHT_FOOT
  STATE MACHINES : MATLAB Function  TreatAsAtomicUnit=on
      settings: PermitHierarchicalResolution=ParametersOnly
  Smooth the Base Pose and send it to the MPC : Subsystem
  checkIMU : Scope
      settings: TimeRange=auto  ShowLegends=on  MaxDataPoints=5000  SaveToWorkspace=off  SaveName=ScopeData3  YMin=-86.69209  YMax=62.14847  SampleTime=-1
  feetInContact (MPC) : WBToolboxLibrary/Utilities/Yarp Read  portName=Ports.ACTIVE_CONTACTS  signalSize=2  timeout=0.5  blocking=off  timestamp=off  autoconnect=on  errorOnConnection=off
  holder 1 : WBToolboxLibrary/Utilities/holder 
  holder 5 : WBToolboxLibrary/Utilities/holder 
  left_foot_wrench : WBToolboxLibrary/Utilities/Yarp Read  portName=Ports.LEFT_FOOT_EXT_WRENCH  signalSize=6  timeout=0.5  blocking=off  timestamp=off  autoconnect=on  errorOnConnection=on
  pos_vel_acc_CoM_des (MPC) : WBToolboxLibrary/Utilities/Yarp Read  portName=Ports.COM_DES  signalSize=9  timeout=0.5  blocking=off  timestamp=off  autoconnect=on  errorOnConnection=off
  right_foot_wrench : WBToolboxLibrary/Utilities/Yarp Read  portName=Ports.RIGHT_FOOT_EXT_WRENCH  signalSize=6  timeout=0.5  blocking=off  timestamp=off  autoconnect=on  errorOnConnection=on
  rotational task : WBToolboxLibrary/wholeBodyModel/Kinematics/Forward Kinematics  frameName=Frames.ROT_TASK_LINK
  s_des (MPC) : WBToolboxLibrary/Utilities/Yarp Read  portName=Ports.Q_DES  signalSize=23  timeout=0.5  blocking=off  timestamp=off  autoconnect=on  errorOnConnection=off
  waistIMU : WBToolboxLibrary/Utilities/Yarp Read  portName='/icub/xsens_inertial'  signalSize=12  timeout=0.5  blocking=off  timestamp=off  autoconnect=on  errorOnConnection=on
  w_H_b : Outport
  feetInContact : Outport  Port=2
  BaseVelocity : Outport  Port=3
  "omega_world " : Outport  Port=4
  state : Outport  Port=5
  references_CoM : Outport  Port=6
  references_LFoot : Outport  Port=7
  references_RFoot : Outport  Port=8
  references_rot_task : Outport  Port=9
  references_s : Outport  Port=10
  leftIsFixed : Outport  Port=11
  useFeetPIDs : Outport  Port=12
  tag scope: feetInContactMPC=global, leftIsFixed=global, useFeetPIDs=global, w_H_b=global, w_H_bWithIMu=global
  wires:
  s/1 -> RFoot to world transform (fixed base)/2, rotational task/2, holder 5/1
  w_walking_H_b_initial/1 -> rotational task/1
  ON_GAZEBO 3/1 -> Emergency Stop/Enable
  STATE MACHINES/10(leftIsFixed_out) -> [leftIsFixed], leftIsFixed/1
  holder 5/1 -> STATE MACHINES/1(s_0)
  rotational task/1 -> holder 1/1
  holder 1/1 -> STATE MACHINES/2(w_H_rot_task_initial)
  w_walking_H_LFoot/1 -> STATE MACHINES/3(w_walking_H_LFoot)
  w_walking_H_RFoot/1 -> STATE MACHINES/4(w_walking_H_RFoot)
  b_H_RFoot/1 -> STATE MACHINES/6(b_H_RFoot)
  b_H_LFoot/1 -> STATE MACHINES/5(b_H_LFoot)
  LFoot_is_fixed (MPC)/1 -> STATE MACHINES/8(LFoot_is_fixed)
  pos_vel_acc_CoM_des (MPC)/1 -> Emergency Stop/1(CoM_des), STATE MACHINES/9(pos_vel_acc_CoM_des_walking)
  s_des (MPC)/1 -> STATE MACHINES/10(s_des_walking)
  left_foot_wrench/1 -> STATE MACHINES/12(LFoot_wrench)
  right_foot_wrench/1 -> STATE MACHINES/13(RFoot_wrench)
  STATE MACHINES/1(state) -> state/1
  STATE MACHINES/2(references_CoM) -> references_CoM/1
  STATE MACHINES/3(references_LFoot) -> references_LFoot/1
  STATE MACHINES/4(references_RFoot) -> references_RFoot/1
  STATE MACHINES/5(references_rot_task) -> references_rot_task/1
  STATE MACHINES/6(feetInContact) -> feetInContact/1
  STATE MACHINES/7(references_s) -> references_s/1
  feetInContact (MPC)/1 -> [feetInContactMPC], STATE MACHINES/11(feetInContact_walking)
  Smooth the Base Pose and send it to the MPC/1(w_H_b_smoothed) -> w_H_b/1
  STATE MACHINES/11(useFeetPIDs) -> [useFeetPIDs], useFeetPIDs/1
  Smooth the Base Pose and send it to the MPC/2(BaseVelocity) -> BaseVelocity/1
  STATE MACHINES/9(w_H_bWithImu) -> Smooth the Base Pose and send it to the MPC/1(w_H_b), [w_H_bWithIMu]
  Constant/1 -> RFoot to world transform (fixed base)/1
  RFoot to world transform (fixed base)/1 -> STATE MACHINES/7(b_H_RFoot_desired)
  waistIMU/1 -> checkIMU/1, STATE MACHINES/14(waistImu)
  STATE MACHINES/8(w_H_b) -> [w_H_b]
  STATE MACHINES/12(omega_world) -> "omega_world "/1

== system taskBasedWalking_legacy/Visualization/Visualize Cartesian Tasks/Rotation Error Left Foot ==
  w_R_LFoot : Inport
  w_R_LFoot_des : Inport  Port=2
  Permute Dimensions2 : PermuteDimensions
  Product2 : Product  Multiplication=Matrix(*)
  Rot error using roll-pitch-yaw : MATLAB Function  TreatAsAtomicUnit=on
      settings: PermitHierarchicalResolution=ParametersOnly
  rollPitchYaw : Outport
  wires:
  w_R_LFoot_des/1 -> Product2/2
  w_R_LFoot/1 -> Permute Dimensions2/1
  Permute Dimensions2/1 -> Product2/1
  Rot error using roll-pitch-yaw/1(rollPitchYaw) -> rollPitchYaw/1
  Product2/1 -> Rot error using roll-pitch-yaw/1(R_0)

== system taskBasedWalking_legacy/Visualization/Visualize Cartesian Tasks/Rotation Error Right Foot ==
  w_R_RFoot : Inport
  w_R_RFoot_des : Inport  Port=2
  Permute Dimensions2 : PermuteDimensions
  Product2 : Product  Multiplication=Matrix(*)
  Rot error using roll-pitch-yaw : MATLAB Function  TreatAsAtomicUnit=on
      settings: PermitHierarchicalResolution=ParametersOnly
  rollPitchYaw : Outport
  wires:
  w_R_RFoot_des/1 -> Product2/2
  w_R_RFoot/1 -> Permute Dimensions2/1
  Permute Dimensions2/1 -> Product2/1
  Rot error using roll-pitch-yaw/1(rollPitchYaw) -> rollPitchYaw/1
  Product2/1 -> Rot error using roll-pitch-yaw/1(R_0)

== system taskBasedWalking_legacy/Visualization/Visualize Cartesian Tasks/Rotation Error Rot Task ==
  w_R_rot_task : Inport
  w_R_rot_task_des : Inport  Port=2
  Permute Dimensions2 : PermuteDimensions
  Product2 : Product  Multiplication=Matrix(*)
  Rot error using roll-pitch-yaw : MATLAB Function  TreatAsAtomicUnit=on
      settings: PermitHierarchicalResolution=ParametersOnly
  rollPitchYaw : Outport
  wires:
  w_R_rot_task_des/1 -> Product2/2
  w_R_rot_task/1 -> Permute Dimensions2/1
  Permute Dimensions2/1 -> Product2/1
  Rot error using roll-pitch-yaw/1(rollPitchYaw) -> rollPitchYaw/1
  Product2/1 -> Rot error using roll-pitch-yaw/1(R_0)

== system taskBasedWalking_legacy/Visualization/Visualize Joints and Floating Base State/Rotation Error Base ==
  w_R_Base : Inport
  Rot error using roll-pitch-yaw : MATLAB Function  TreatAsAtomicUnit=on
      settings: PermitHierarchicalResolution=ParametersOnly
  rollPitchYaw : Outport
  wires:
  Rot error using roll-pitch-yaw/1(rollPitchYaw) -> rollPitchYaw/1
  w_R_Base/1 -> Rot error using roll-pitch-yaw/1(R_0)

== system taskBasedWalking_legacy/Visualization/Visualize Joints and Floating Base State/Rotation Error Base1 ==
  w_R_Base : Inport
  Rot error using roll-pitch-yaw : MATLAB Function  TreatAsAtomicUnit=on
      settings: PermitHierarchicalResolution=ParametersOnly
  rollPitchYaw : Outport
  wires:
  Rot error using roll-pitch-yaw/1(rollPitchYaw) -> rollPitchYaw/1
  w_R_Base/1 -> Rot error using roll-pitch-yaw/1(R_0)

== system taskBasedWalking_legacy/Visualization/Visualize Smoothing (orientation)/Rotation Error Left Foot ==
  w_R_LFoot : Inport
  w_R_LFoot_des : Inport  Port=2
  Permute Dimensions2 : PermuteDimensions
  Product2 : Product  Multiplication=Matrix(*)
  Rot error using roll-pitch-yaw : MATLAB Function  TreatAsAtomicUnit=on
      settings: PermitHierarchicalResolution=ParametersOnly
  rollPitchYaw : Outport
  wires:
  w_R_LFoot_des/1 -> Product2/2
  w_R_LFoot/1 -> Permute Dimensions2/1
  Permute Dimensions2/1 -> Product2/1
  Rot error using roll-pitch-yaw/1(rollPitchYaw) -> rollPitchYaw/1
  Product2/1 -> Rot error using roll-pitch-yaw/1(R_0)

== system taskBasedWalking_legacy/Visualization/Visualize Smoothing (orientation)/Rotation Error Right Foot ==
  w_R_RFoot : Inport
  w_R_RFoot_des : Inport  Port=2
  Permute Dimensions2 : PermuteDimensions
  Product2 : Product  Multiplication=Matrix(*)
  Rot error using roll-pitch-yaw : MATLAB Function  TreatAsAtomicUnit=on
      settings: PermitHierarchicalResolution=ParametersOnly
  rollPitchYaw : Outport
  wires:
  w_R_RFoot_des/1 -> Product2/2
  w_R_RFoot/1 -> Permute Dimensions2/1
  Permute Dimensions2/1 -> Product2/1
  Rot error using roll-pitch-yaw/1(rollPitchYaw) -> rollPitchYaw/1
  Product2/1 -> Rot error using roll-pitch-yaw/1(R_0)

== system taskBasedWalking_legacy/Visualization/Visualize Smoothing (orientation)/Rotation Error Rot Task ==
  w_R_rot_task : Inport
  w_R_rot_task_des : Inport  Port=2
  Permute Dimensions2 : PermuteDimensions
  Product2 : Product  Multiplication=Matrix(*)
  Rot error using roll-pitch-yaw : MATLAB Function  TreatAsAtomicUnit=on
      settings: PermitHierarchicalResolution=ParametersOnly
  rollPitchYaw : Outport
  wires:
  w_R_rot_task_des/1 -> Product2/2
  w_R_rot_task/1 -> Permute Dimensions2/1
  Permute Dimensions2/1 -> Product2/1
  Rot error using roll-pitch-yaw/1(rollPitchYaw) -> rollPitchYaw/1
  Product2/1 -> Rot error using roll-pitch-yaw/1(R_0)

== system taskBasedWalking_legacy/Dynamics and Kinematics/Compute Dynamic and Kinematic Quantities/Mass Matrix and Bias Forces/Add motors reflected inertias ==
  M : Inport
  Add motor reflected inertias : MATLAB Function  TreatAsAtomicUnit=on
      settings: PermitHierarchicalResolution=ParametersOnly
  M_with_motor_inertia : Outport
  wires:
  M/1 -> Add motor reflected inertias/1(M)
  Add motor reflected inertias/1(M_with_inertia) -> M_with_motor_inertia/1

== system taskBasedWalking_legacy/Dynamics and Kinematics/Compute Tasks Accelerations/ComputeTasksPoseAndVelocity/Task position and orientation ==
  s : Inport
  w_H_b : Inport  Port=2
  CoM : WBToolboxLibrary/wholeBodyModel/Kinematics/Forward Kinematics  frameName=Frames.COM
  LFoot : WBToolboxLibrary/wholeBodyModel/Kinematics/Forward Kinematics  frameName=Frames.LEFT_FOOT
  RFoot : WBToolboxLibrary/wholeBodyModel/Kinematics/Forward Kinematics  frameName=Frames.RIGHT_FOOT
  rotational task : WBToolboxLibrary/wholeBodyModel/Kinematics/Forward Kinematics  frameName=Frames.ROT_TASK_LINK
  w_H_CoM : Outport
  w_H_l_sole : Outport  Port=2
  w_H_r_sole : Outport  Port=3
  w_H_rot_task : Outport  Port=4
  wires:
  s/1 -> rotational task/2, RFoot/2, LFoot/2, CoM/2
  w_H_b/1 -> rotational task/1, CoM/1, LFoot/1, RFoot/1
  CoM/1 -> w_H_CoM/1
  LFoot/1 -> w_H_l_sole/1
  RFoot/1 -> w_H_r_sole/1
  rotational task/1 -> w_H_rot_task/1

== system taskBasedWalking_legacy/Robot State and References/Smooth References /Smooth Reference Orientations/Compose Smoothed References ==
  omegaDot_LFoot : Inport
  omegaDot_RFoot : Inport  Port=2
  omegaDot_rot_task : Inport  Port=3
  w_R_rot_task : Inport  Port=4
  w_R_RFoot : Inport  Port=5
  w_R_LFoot : Inport  Port=6
  omega_LFoot : Inport  Port=7
  omega_RFoot : Inport  Port=8
  omega_rot_task : Inport  Port=9
  Matrix Concatenate1 : Concatenate  NumInputs=3  Mode=Multidimensional array  ConcatenateDimension=2
  Matrix Concatenate2 : Concatenate  NumInputs=3  Mode=Multidimensional array  ConcatenateDimension=2
  Matrix Concatenate6 : Concatenate  NumInputs=3  Mode=Multidimensional array  ConcatenateDimension=2
  orient_vel_acc_LFoot_des : Outport
  orient_vel_acc_RFoot_des : Outport  Port=2
  orient_vel_acc_rot_task_des : Outport  Port=3
  wires:
  w_R_LFoot/1 -> Matrix Concatenate6/1
  Matrix Concatenate6/1 -> orient_vel_acc_LFoot_des/1
  Matrix Concatenate2/1 -> orient_vel_acc_rot_task_des/1
  Matrix Concatenate1/1 -> orient_vel_acc_RFoot_des/1
  omega_LFoot/1 -> Matrix Concatenate6/2
  omega_RFoot/1 -> Matrix Concatenate1/2
  w_R_RFoot/1 -> Matrix Concatenate1/1
  omega_rot_task/1 -> Matrix Concatenate2/2
  w_R_rot_task/1 -> Matrix Concatenate2/1
  omegaDot_LFoot/1 -> Matrix Concatenate6/3
  omegaDot_RFoot/1 -> Matrix Concatenate1/3
  omegaDot_rot_task/1 -> Matrix Concatenate2/3
